simulink model "f18trim"  (R2017a)
settings: Solver=ode45  StartTime=0.0  StopTime=10.0  RelTol=1e-3  EnableMultiTasking=on
settings Model: Creator=mpc5200  LastModifiedBy=Gaurav Misra
settings DataIOCC: LimitDataPoints=on  SaveFormat=Array  SignalLoggingSaveFormat=ModelDataLogs
settings OptimizationCC: ExpressionDepthLimit=2147483647  InitFltsAndDblsToZero=on  LifeSpan=inf
settings DebuggingCC: AlgebraicLoopMsg=none  SaveWithParameterizedLinksMsg=none  UnderspecifiedInitializationDetection=Classic  MergeDetectMultiDrivingBlocksExec=none  FcnCallInpInsideContextMsg=warning  UnconnectedInputMsg=none  UnconnectedOutputMsg=none  UnconnectedLineMsg=none  StateNameClashWarn=warning  SFUnexpectedBacktrackingDiag=warning  SFNoUnconditionalDefaultTransitionDiag=warning  SFExecutionAtInitializationDiag=none
settings HardwareCC: ProdBitPerPointer=32  ProdBitPerSizeT=32  ProdBitPerPtrDiffT=32  ProdLargestAtomicFloat=None  ProdIntDivRoundTo=Undefined  ProdEndianess=Unspecified  ProdWordSize=32  ProdHWDeviceType=32-bit Generic
settings ModelReferenceCC: PropagateSignalLabelsOutOfModel=off
settings GRTTargetCC: TargetFcnLib=ansi_tfl_tmw.mat  TargetLangStandard=C89/C90 (ANSI)  CombineOutputUpdateFcns=off  GRTInterface=on
settings ConfigComp: CovMetricSettings=dw  CovHtmlReporting=on  CovSaveCumulativeToWorkspaceVar=on  CovSaveSingleToWorkspaceVar=on  CovExternalEMLEnable=off

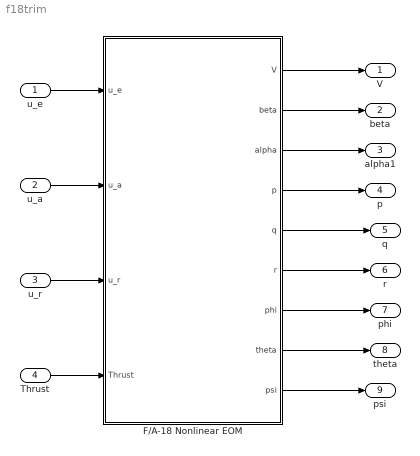
== system f18trim ==
  u_e : Inport
  u_a : Inport  Port=2
  u_r : Inport  Port=3
  Thrust : Inport  Port=4
  F/A-18 Nonlinear EOM : Subsystem
  V : Outport
  beta : Outport  Port=2
  alpha1 : Outport  Port=3
  p : Outport  Port=4
  q : Outport  Port=5
  r : Outport  Port=6
  phi : Outport  Port=7
  theta : Outport  Port=8
  psi : Outport  Port=9
  wires:
  F/A-18 Nonlinear EOM/1(V) -> V/1
  F/A-18 Nonlinear EOM/2(beta) -> beta/1
  F/A-18 Nonlinear EOM/3(alpha) -> alpha1/1
  F/A-18 Nonlinear EOM/4(p) -> p/1
  F/A-18 Nonlinear EOM/5(q) -> q/1
  F/A-18 Nonlinear EOM/6(r) -> r/1
  F/A-18 Nonlinear EOM/8(theta) -> theta/1
  u_a/1 -> F/A-18 Nonlinear EOM/2(u_a)
  F/A-18 Nonlinear EOM/9(psi) -> psi/1
  F/A-18 Nonlinear EOM/7(phi) -> phi/1
  u_r/1 -> F/A-18 Nonlinear EOM/3(u_r)
  Thrust/1 -> F/A-18 Nonlinear EOM/4(Thrust)
  u_e/1 -> F/A-18 Nonlinear EOM/1(u_e)

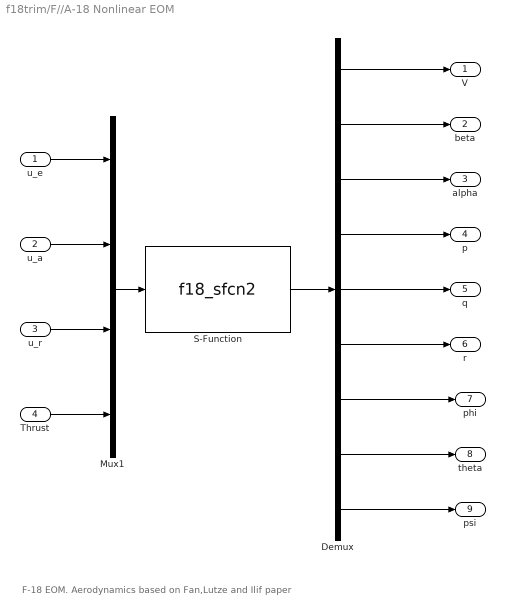
== system f18trim/F//A-18 Nonlinear EOM ==
  note: F-18 EOM. Aerodynamics based on Fan,Lutze and Ilif paper
  u_e : Inport
  u_a : Inport  Port=2
  u_r : Inport  Port=3
  Thrust : Inport  Port=4
  Demux : Demux  Outputs=9
  Mux1 : Mux
  S-Function : S-Function  FunctionName=f18_sfcn2  Parameters=x0  SFunctionDeploymentMode=off  EnableBusSupport=off
  V : Outport
  beta : Outport  Port=2
  alpha : Outport  Port=3
  p : Outport  Port=4
  q : Outport  Port=5
  r : Outport  Port=6
  phi : Outport  Port=7
  theta : Outport  Port=8
  psi : Outport  Port=9
  wires:
  Mux1/1 -> S-Function/1
  S-Function/1 -> Demux/1
  Demux/1 -> V/1
  Demux/5 -> q/1
  Demux/2 -> beta/1
  Demux/3 -> alpha/1
  Demux/4 -> p/1
  Demux/6 -> r/1
  Demux/7 -> phi/1
  Demux/8 -> theta/1
  Demux/9 -> psi/1
  u_r/1 -> Mux1/3
  Thrust/1 -> Mux1/4
  u_a/1 -> Mux1/2
  u_e/1 -> Mux1/1
